simulink model "model_2_1"  (R2021b)
settings: Solver=FixedStepAuto  StartTime=0.0  StopTime=5  FixedStep=0.00005  RelTol=1e-3
settings Model: Creator=den  LastModifiedBy=den

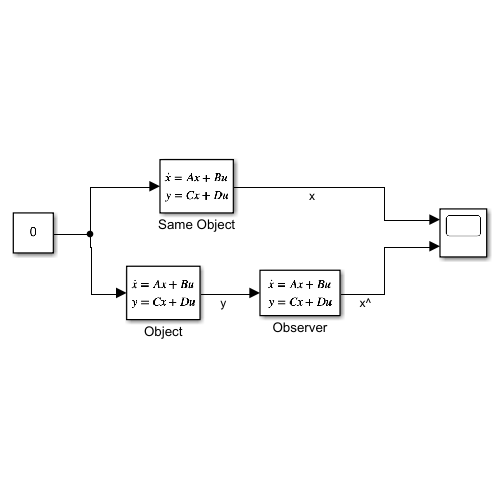
[thumbnail: Simulink's stored preview of the top-level diagram]
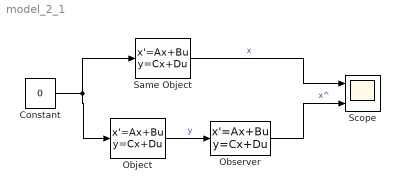
== system model_2_1 ==
  Constant : Constant  Value=0
  Object : StateSpace  A=[0 5 0 0; -5 0 0 0; 0 0 0 1; 0 0 -1 0]  B=[0; 0; 0; 0]  C=[0 9 1 0]  D=0  InitialCondition=[1;1;1;1]
  Observer : StateSpace  A=[0 10.3667 0.596296 0; -5 -8 -0.88889 0; 0 -36 -4 1; 0 -10.5 -2.166667 0]  B=[-0.596296; 0.88889; 4; 1.16667]  C=[1 0 0 0; 0 1 0 0; 0 0 1 0; 0 0 0 1]  D=[0;0;0;0]  InitialCondition=[2;0;0;-1]
  Same Object : StateSpace  A=[0 5 0 0; -5 0 0 0; 0 0 0 1; 0 0 -1 0]  B=[0; 0; 0; 0]  C=[1 0 0 0; 0 1 0 0; 0 0 1 0; 0 0 0 1]  D=[0;0;0;0]  InitialCondition=[1;1;1;1]
  Scope : Scope  NumInputPorts=2
  wires:
  Object/1 -> Observer/1  "y"
  Observer/1 -> Scope/2  "x^"
  Constant/1 -> Object/1, Same Object/1
  Same Object/1 -> Scope/1  "x"
